simulink model "LinearInvertedPendulum"  (R2017a)
settings: Solver=VariableStepAuto  StartTime=0.0  StopTime=600.0  RelTol=1e-3
values from neighbouring files (symbols this model uses):
  A_a = double(subs(A_a, [x1, x2, x3, x4, u], [x10, x20, x30, x40, u0]))    [Inverted_pendulum.m]
  b = 0.1    [Inverted_pendulum.m]
  B_a = double(subs(B_a, [x1, x2, x3, x4, u], [x10, x20, x30, x40, u0]))    [Inverted_pendulum.m]
  C_a = double(subs(C_a, [x1, x2, x3, x4, u], [x10, x20, x30, x40, u0]))    [Inverted_pendulum.m]
  D_a = [0 ; 0]    [Inverted_pendulum.m]
  g = 9.8    [Inverted_pendulum.m]
  I = 0.006    [Inverted_pendulum.m]
  L = 0.3    [Inverted_pendulum.m]
  M = 0.5    [Inverted_pendulum.m]    (also in jury.m = vpa(M))
  u0 = double(equilibrium.u(n))    [Inverted_pendulum.m]
  x10 = double(equilibrium.x1(n))    [Inverted_pendulum.m]
  x30 = double(equilibrium.x3(n))    [Inverted_pendulum.m]
undefined symbols (not defined in the file): m, x20, x40
settings Model: Creator=aposad31  LastModifiedBy=Asus

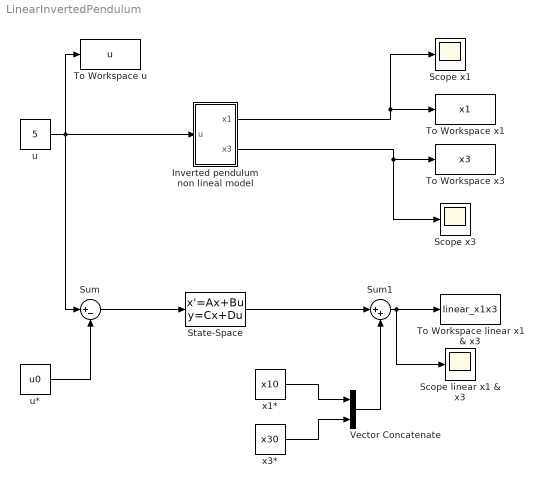
== system LinearInvertedPendulum ==
  Inverted pendulum non lineal model : Subsystem  mask{M=M, m_p=m, b=b, I=I, L=L, g=g, dx10=x10, dx20=x20, dx30=x30, dx40=x40}
      mask prompts: m_p "m"
      mask TypeOptions M: M/Value
      mask TypeOptions m_p: m/Value
      mask TypeOptions b: b/Value
      mask TypeOptions I: I/Value
      mask TypeOptions L: L/Value
      mask TypeOptions g: g/Value
      mask TypeOptions dx10: dx1/InitialCondition
      mask TypeOptions dx20: dx2/InitialCondition
      mask TypeOptions dx30: dx3/InitialCondition
      mask TypeOptions dx40: dx4/InitialCondition
      mask DialogControl Initial_conditions Prompt: Initial conditions
  Scope linear x1 & x3 : Scope
  Scope x1 : Scope
  Scope x3 : Scope
  State-Space : StateSpace  A=A_a  B=B_a  C=C_a  D=D_a  X0=0
  Sum : Sum  Inputs=|+-
  Sum1 : Sum  Inputs=|++
  To Workspace linear x1 & x3 : ToWorkspace  VariableName=linear_x1x3  SaveFormat=Timeseries  SampleTime=-1
  To Workspace u : ToWorkspace  VariableName=u  SaveFormat=Timeseries  SampleTime=-1
  To Workspace x1 : ToWorkspace  VariableName=x1  SaveFormat=Timeseries  SampleTime=-1
  To Workspace x3 : ToWorkspace  VariableName=x3  SaveFormat=Timeseries  SampleTime=-1
  Vector Concatenate : Concatenate
  u : Constant  Value=5
  u* : Constant  Value=u0
  x1* : Constant  Value=x10
  x3* : Constant  Value=x30
  wires:
  u/1 -> To Workspace u/1, Sum/1, Inverted pendulum non lineal model/1(u)
  Inverted pendulum non lineal model/1(x1) -> Scope x1/1, To Workspace x1/1
  Inverted pendulum non lineal model/2(x3) -> Scope x3/1, To Workspace x3/1
  u*/1 -> Sum/2
  Sum/1 -> State-Space/1
  x1*/1 -> Vector Concatenate/1
  x3*/1 -> Vector Concatenate/2
  Vector Concatenate/1 -> Sum1/2
  State-Space/1 -> Sum1/1
  Sum1/1 -> Scope linear x1 & x3/1, To Workspace linear x1 & x3/1

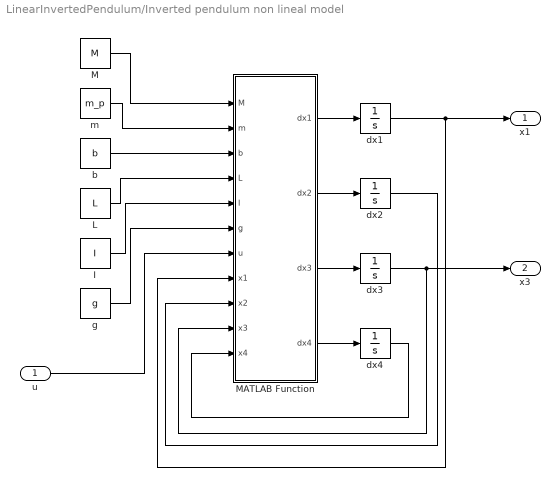
== system LinearInvertedPendulum/Inverted pendulum non lineal model ==
  u : Inport
  I : Constant  Value=I
  L : Constant  Value=L
  M : Constant  Value=M
  MATLAB Function : MATLAB Function  TreatAsAtomicUnit=on
  b : Constant  Value=b
  dx1 : Integrator  InitialCondition=dx10
  dx2 : Integrator  InitialCondition=dx20
  dx3 : Integrator  InitialCondition=dx30
  dx4 : Integrator  InitialCondition=dx40
  g : Constant  Value=g
  m : Constant  Value=m_p
  x1 : Outport
  x3 : Outport  Port=2
  wires:
  MATLAB Function/2(dx2) -> dx2/1
  g/1 -> MATLAB Function/6(g)
  MATLAB Function/4(dx4) -> dx4/1
  M/1 -> MATLAB Function/1(M)
  MATLAB Function/1(dx1) -> dx1/1
  u/1 -> MATLAB Function/7(u)
  m/1 -> MATLAB Function/2(m)
  I/1 -> MATLAB Function/5(I)
  dx4/1 -> MATLAB Function/11(x4)
  MATLAB Function/3(dx3) -> dx3/1
  dx2/1 -> MATLAB Function/9(x2)
  b/1 -> MATLAB Function/3(b)
  dx1/1 -> x1/1, MATLAB Function/8(x1)
  L/1 -> MATLAB Function/4(L)
  dx3/1 -> x3/1, MATLAB Function/10(x3)

== matlab function LinearInvertedPendulum/Inverted pendulum non lineal model/MATLAB Function ==
  data: M input; m input; b input; L input; I input; g input; u input; dx1 output; x1 input; x2 input; x3 input; x4 input; dx2 output; dx3 output; dx4 output
function [dx1, dx2, dx3, dx4] = fcn(M, m, b, L, I, g, u, x1, x2, x3, x4)
    denominator = (M+m)*(I+m*L^2)-m^2*L^2*cos(x3)^2;
    dx1 = x2;
    dx2 = ((I+m*L^2)*(u-b*x2+m*L*x4^2*sin(x3))+m^2*L^2*g*sin(x3)*cos(x3))/denominator;
    dx3 = x4;
    dx4 = (-m*L*u*cos(x3)+m*L*b*x2*cos(x3)-m^2*L^2*x4^2*sin(x3)*cos(x3)-(M+m)*m*g*L*sin(x3))/denominator;
end
